simulink model "point_Dynamics_a"  (R2018a)
settings: Solver=ode45  StartTime=0.0  StopTime=30  RelTol=1e-6  AbsTol=1e-6
values from neighbouring files (symbols this model uses):
  cableLength = quadrotor.ell    [initSim.m]
  gravity = quadrotor.g    [initSim.m]
  initQuadPos = [1 1 -2]'    [initSim.m]
  loadMass = quadrotor.m    [initSim.m]    (also in quadrotor_dynamics_extended.m = quad.loadMass)
  maxCargoWeight = quadrotor.M/2    [initSim.m]
  quadMass = quadrotor.M    [initSim.m]
  tensionLowerBound = 0.1    [initSim.m]
  tensionUpperBound = 0.1    [initSim.m]
undefined symbols (not defined in the file or in its folder): quadrotor
settings Model: Creator=Henrik  LastModifiedBy=Henrik
settings SolverCC: AutoScaleAbsTol=off  ShapePreserveControl=EnableAll

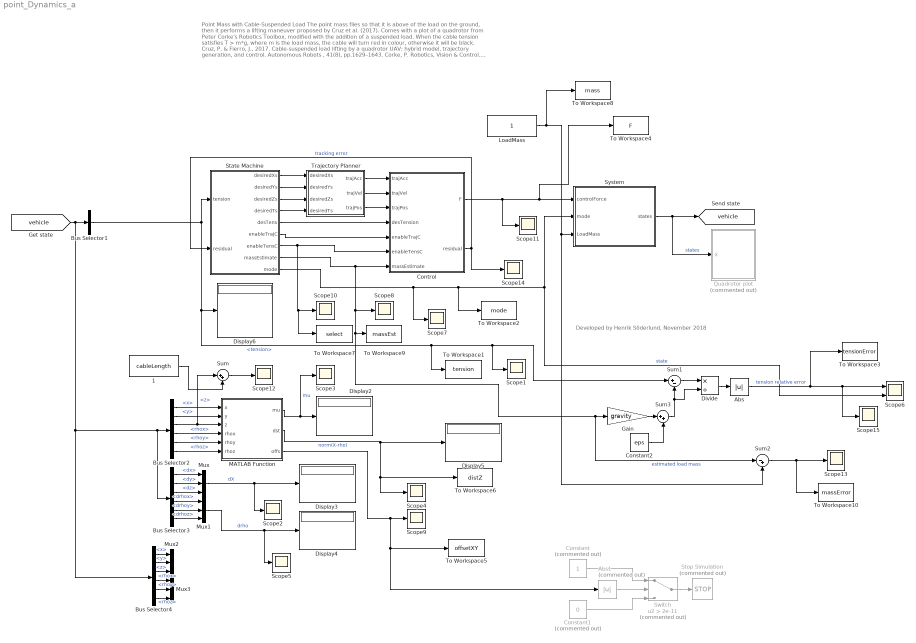
== system point_Dynamics_a ==
  note: Point Mass with Cable-Suspended Load
      |
      | The point mass flies so that it is above of the load on the ground, then it performs a lifting maneuver proposed by Cruz et al. (2017).
      |
      | Comes with a plot of a quadrotor from Peter Corke's Robotics Toolbox, modified with the addition of a suspended load. When the cable tension satisfies T > m*g, where m is the load mass, the cable will turn red in colour, otherwise it will be black.
      |
      | Cruz, P. & Fierro, J., 2017. Cable-suspended load lifting by a quadrotor UAV: hybrid model, trajectory generation, and control. Autonomous Robots , 41(8), pp.1629–1643.
      |
      | Corke, P. Robotics, Vision & Control. Springer (2017).
  note: Developed by Henrik Söderlund, November 2018
  1 : Constant  Value=cableLength
  Abs : Abs
  Abs1 : Abs  Commented=on
  Bus Selector1 : BusSelector  OutputSignals=tension
  Bus Selector2 : BusSelector  OutputSignals=x,y,z,rhox,rhoy,rhoz
  Bus Selector3 : BusSelector  OutputSignals=dx,dy,dz,drhox,drhoy,drhoz
  Bus Selector4 : BusSelector  OutputSignals=x,y,z,rhox,rhoy,rhoz
  Constant : Constant  Commented=on
  Constant1 : Constant  Commented=on  Value=0
  Constant2 : Constant  Value=eps
  Control : Subsystem
  Display{2..6} (5 alike) : Display
  Divide : Product  Inputs=*/
  Gain : Gain  Gain=gravity
  LoadMass : Constant
  MATLAB Function : MATLAB Function  TreatAsAtomicUnit=on
  Mux{,1..3} (4 alike) : Mux  Inputs=3
  Quadrotor plot : Subsystem  Commented=on  AncestorBlock=roblocks/Vehicles/Quadrotor plot  mask{quad=quadrotor, xydim=2, zdim=10}
      mask prompts: quad "Model"; xydim "xy-axes dimension"; zdim "z-axis dimension"
      mask help: Animate quadrotor.
      mask Help:
      | This block graphically displays a quadrotor (flying robot).
      | 
      | A new figure is created and A graphical model of a quadrotor is animated
      | to a pose specified by the state vector input to the block.
      | 
      | The state vector is [x y z roll pitch yaw] in world coordinates and the
      | angles are in radians.
      | 
      | Notes:
      | - The dimensions of the vehicle workspace are set by parameters
  Scope{1..5,7..15} (14 alike) : Scope
  Scope6 : Scope  NumInputPorts=2
  State Machine : Subsystem
  Stop Simulation : Stop  Commented=on
  Sum : Sum  Inputs=|++
  Sum1 : Sum  Inputs=|+-
  Sum2 : Sum  Inputs=|-+
  Sum3 : Sum  Inputs=|++
  Switch : Switch  Commented=on  Criteria=u2 > Threshold  Threshold=2e-11
  System : Subsystem
  To Workspace1 : ToWorkspace  VariableName=tension  SaveFormat=Timeseries  SampleTime=-1
      settings: Save2DSignal=2-D array (concatenate along first dimension)
  To Workspace10 : ToWorkspace  VariableName=massError  SaveFormat=Timeseries  SampleTime=-1
      settings: Save2DSignal=2-D array (concatenate along first dimension)
  To Workspace2 : ToWorkspace  VariableName=mode  SaveFormat=Timeseries  SampleTime=-1
      settings: Save2DSignal=2-D array (concatenate along first dimension)
  To Workspace3 : ToWorkspace  VariableName=tensionError  SaveFormat=Timeseries  SampleTime=-1
      settings: Save2DSignal=2-D array (concatenate along first dimension)
  To Workspace4 : ToWorkspace  VariableName=F  SaveFormat=Timeseries  SampleTime=-1
      settings: Save2DSignal=2-D array (concatenate along first dimension)
  To Workspace5 : ToWorkspace  VariableName=offsetXY  SaveFormat=Timeseries  SampleTime=-1
      settings: Save2DSignal=2-D array (concatenate along first dimension)
  To Workspace6 : ToWorkspace  VariableName=distZ  SaveFormat=Timeseries  SampleTime=-1
      settings: Save2DSignal=2-D array (concatenate along first dimension)
  To Workspace7 : ToWorkspace  VariableName=select  SaveFormat=Timeseries  SampleTime=-1
      settings: Save2DSignal=2-D array (concatenate along first dimension)
  To Workspace8 : ToWorkspace  VariableName=mass  SaveFormat=Timeseries  SampleTime=-1
      settings: Save2DSignal=2-D array (concatenate along first dimension)
  To Workspace9 : ToWorkspace  VariableName=massEst  SaveFormat=Timeseries  SampleTime=-1
      settings: Save2DSignal=2-D array (concatenate along first dimension)
  Trajectory Planner : Subsystem
  tag scope: vehicle=global
  wires:
  [vehicle] -> Bus Selector4/1, Bus Selector2/1, Bus Selector3/1, Bus Selector1/1
  Bus Selector1/1 -> To Workspace1/1, Scope1/1, Sum1/1, Display6/1, State Machine/1(tension)  "<tension>"
  State Machine/1(desiredXs) -> Trajectory Planner/1(desiredXs)
  State Machine/2(desiredYs) -> Trajectory Planner/2(desiredYs)
  State Machine/3(desiredZs) -> Trajectory Planner/3(desiredZs)
  State Machine/4(desiredTs) -> Trajectory Planner/4(desiredTs)
  System/1(states) -> Quadrotor plot/1(X), [vehicle]  "states"
  State Machine/9(mode) -> Scope7/1, To Workspace2/1, Scope6/2, System/2(mode)  "state"
  Bus Selector2/1 -> MATLAB Function/1(x)  "<x>"
  Bus Selector2/2 -> MATLAB Function/2(y)  "<y>"
  Bus Selector2/3 -> Sum/1, MATLAB Function/3(z)  "<z>"
  Bus Selector2/4 -> MATLAB Function/4(rhox)  "<rhox>"
  Bus Selector2/5 -> MATLAB Function/5(rhoy)  "<rhoy>"
  Bus Selector2/6 -> MATLAB Function/6(rhoz)  "<rhoz>"
  MATLAB Function/1(mu) -> Scope3/1, Display2/1  "mu"
  Bus Selector3/2 -> Mux/2  "<dy>"
  Bus Selector3/1 -> Mux/1  "<dx>"
  Bus Selector3/3 -> Mux/3  "<dz>"
  Bus Selector3/4 -> Mux1/1  "<drhox>"
  Bus Selector3/5 -> Mux1/2  "<drhoy>"
  Bus Selector3/6 -> Mux1/3  "<drhoz>"
  Mux/1 -> Scope2/1, Display3/1  "dX"
  Mux1/1 -> Scope5/1, Display4/1  "drho"
  MATLAB Function/2(dst) -> To Workspace6/1, Scope4/1, Display5/1  "norm(X-rho)"
  Control/1(F) -> Scope11/1, To Workspace4/1, System/1(controlForce)
  Trajectory Planner/1(trajAcc) -> Control/1(trajAcc)
  Trajectory Planner/2(trajVel) -> Control/2(trajVel)
  Trajectory Planner/3(trajPos) -> Control/3(trajPos)
  State Machine/5(desTens) -> Control/4(desTension)
  State Machine/6(enableTrajC) -> Control/5(enableTrajC)
  State Machine/7(enableTensC) -> To Workspace7/1, Scope10/1, Control/6(enableTensC)
  State Machine/8(massEstimate) -> Sum2/1, Gain/1, To Workspace9/1, Scope8/1, Control/7(massEstimate)  "estimated load mass"
  Sum3/1 -> Divide/2, Sum1/2
  Sum1/1 -> Divide/1
  Divide/1 -> Abs/1
  Abs/1 -> To Workspace3/1, Scope15/1, Scope6/1  "tension relative error"
  MATLAB Function/3(offs) -> Abs1/1, To Workspace5/1, Scope9/1
  LoadMass/1 -> To Workspace8/1, Sum2/2, System/3(LoadMass)
  Sum/1 -> Scope12/1
  1/1 -> Sum/2
  Control/2(residual) -> Scope14/1, State Machine/2(residual)  "tracking error"
  Sum2/1 -> To Workspace10/1, Scope13/1
  Bus Selector4/1 -> Mux2/1  "<x>"
  Bus Selector4/2 -> Mux2/2  "<y>"
  Bus Selector4/3 -> Mux2/3  "<z>"
  Bus Selector4/5 -> Mux3/2  "<rhoy>"
  Bus Selector4/6 -> Mux3/3  "<rhoz>"
  Bus Selector4/4 -> Mux3/1  "<rhox>"
  Switch/1 -> Stop Simulation/1
  Abs1/1 -> Switch/2
  Constant/1 -> Switch/1
  Constant1/1 -> Switch/3
  Gain/1 -> Sum3/1
  Constant2/1 -> Sum3/2

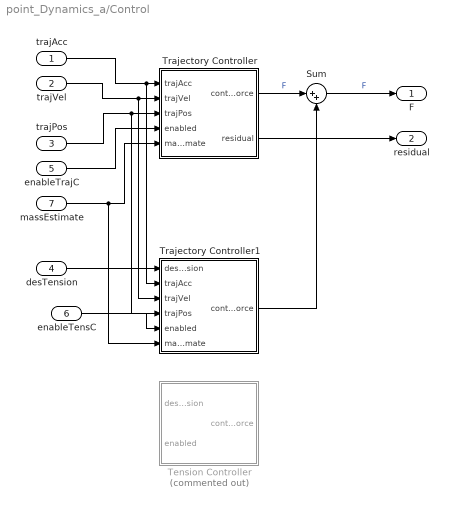
== system point_Dynamics_a/Control ==
  trajAcc : Inport
  trajVel : Inport  Port=2
  trajPos : Inport  Port=3
  desTension : Inport  Port=4
  enableTrajC : Inport  Port=5
  enableTensC : Inport  Port=6
  massEstimate : Inport  Port=7
  Sum : Sum  Inputs=|++
  Tension Controller : Subsystem  Commented=on
  Trajectory Controller : Subsystem
  Trajectory Controller1 : Subsystem
  F : Outport
  residual : Outport  Port=2
  wires:
  Sum/1 -> F/1  "F"
  trajVel/1 -> Trajectory Controller1/3(trajVel), Trajectory Controller/2(trajVel)
  trajPos/1 -> Trajectory Controller1/4(trajPos), Trajectory Controller/3(trajPos)
  enableTrajC/1 -> Trajectory Controller/4(enabled)
  Trajectory Controller/1(controlForce) -> Sum/1  "F"
  trajAcc/1 -> Trajectory Controller1/2(trajAcc), Trajectory Controller/1(trajAcc)
  massEstimate/1 -> Trajectory Controller1/6(massEstimate), Trajectory Controller/5(massEstimate)
  enableTensC/1 -> Trajectory Controller1/5(enabled)
  Trajectory Controller1/1(controlForce) -> Sum/2
  desTension/1 -> Trajectory Controller1/1(desTension)
  Trajectory Controller/2(residual) -> residual/1

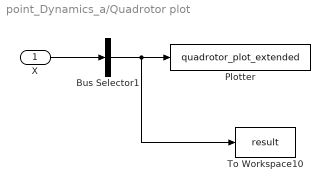
== system point_Dynamics_a/Quadrotor plot ==
  X : Inport
  Bus Selector1 : BusSelector  OutputSignals=x,y,z,yaw,pitch,roll,rhox,rhoy,rhoz,tension  OutputAsBus=on
  Plotter : S-Function  FunctionName=quadrotor_plot_extended  Parameters=[xydim, zdim], 1, 1,quad  SFunctionDeploymentMode=off  EnableBusSupport=off
  To Workspace10 : ToWorkspace  VariableName=result  SampleTime=-1
      settings: Save2DSignal=2-D array (concatenate along first dimension)
  wires:
  X/1 -> Bus Selector1/1
  Bus Selector1/1 -> To Workspace10/1, Plotter/1

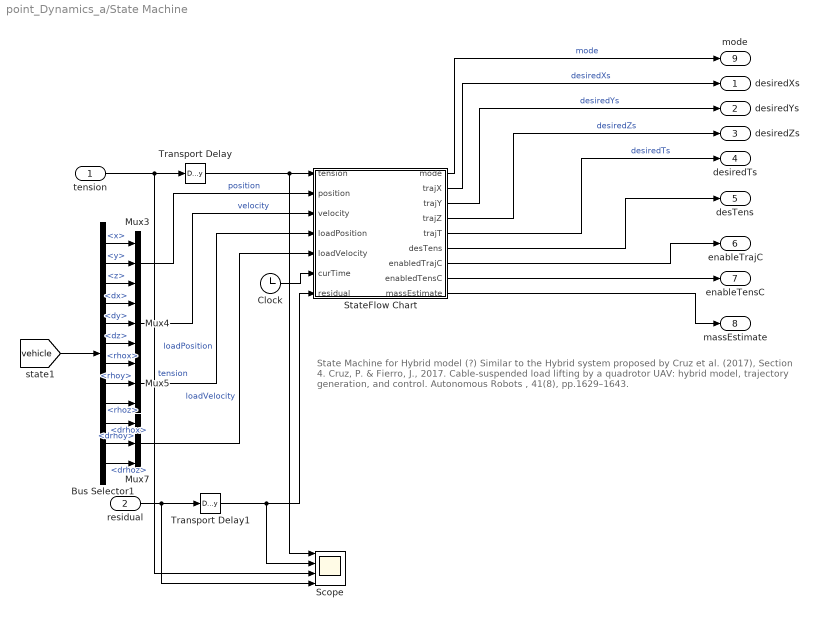
== system point_Dynamics_a/State Machine ==
  note: State Machine for Hybrid model (?)
      |
      | Similar to the Hybrid system proposed by Cruz et al. (2017), Section 4.
      |
      | Cruz, P. & Fierro, J., 2017. Cable-suspended load lifting by a quadrotor UAV: hybrid model, trajectory generation, and control. Autonomous Robots , 41(8), pp.1629–1643.
  tension : Inport
  residual : Inport  Port=2
  Bus Selector1 : BusSelector  OutputSignals=x,y,z,dx,dy,dz,rhox,rhoy,rhoz,drhox,drhoy,drhoz
  Clock : Clock
  Mux{3..5,7} (4 alike) : Mux  Inputs=3
  Scope : Scope  NumInputPorts=4
  StateFlow Chart : Stateflow chart  TreatAsAtomicUnit=on
  Transport Delay : TransportDelay  DelayTime=0.001
  Transport Delay1 : TransportDelay  DelayTime=0.001
  desiredXs : Outport
  desiredYs : Outport  Port=2
  desiredZs : Outport  Port=3
  desiredTs : Outport  Port=4
  desTens : Outport  Port=5
  enableTrajC : Outport  Port=6
  enableTensC : Outport  Port=7
  massEstimate : Outport  Port=8
  mode : Outport  Port=9
  wires:
  StateFlow Chart/5(trajT) -> desiredTs/1  "desiredTs"
  Bus Selector1/1 -> Mux3/1  "<x>"
  Mux3/1 -> StateFlow Chart/2(position)  "position"
  Mux4/1 -> StateFlow Chart/3(velocity)  "velocity"
  Bus Selector1/2 -> Mux3/2  "<y>"
  Mux5/1 -> StateFlow Chart/4(loadPosition)  "loadPosition"
  StateFlow Chart/1(mode) -> mode/1  "mode"
  [vehicle] -> Bus Selector1/1
  Mux7/1 -> StateFlow Chart/5(loadVelocity)  "loadVelocity"
  Bus Selector1/3 -> Mux3/3  "<z>"
  Bus Selector1/7 -> Mux5/1  "<rhox>"
  Bus Selector1/8 -> Mux5/2  "<rhoy>"
  Bus Selector1/9 -> Mux5/3  "<rhoz>"
  Bus Selector1/5 -> Mux4/2  "<dy>"
  Bus Selector1/6 -> Mux4/3  "<dz>"
  Bus Selector1/4 -> Mux4/1  "<dx>"
  Bus Selector1/11 -> Mux7/2  "<drhoy>"
  Bus Selector1/10 -> Mux7/1  "<drhox>"
  Bus Selector1/12 -> Mux7/3  "<drhoz>"
  StateFlow Chart/2(trajX) -> desiredXs/1  "desiredXs"
  StateFlow Chart/4(trajZ) -> desiredZs/1  "desiredZs"
  StateFlow Chart/3(trajY) -> desiredYs/1  "desiredYs"
  tension/1 -> Transport Delay/1, Scope/3  "tension"
  StateFlow Chart/6(desTens) -> desTens/1
  StateFlow Chart/7(enabledTrajC) -> enableTrajC/1
  StateFlow Chart/8(enabledTensC) -> enableTensC/1
  Transport Delay/1 -> Scope/1, StateFlow Chart/1(tension)
  Clock/1 -> StateFlow Chart/6(curTime)
  StateFlow Chart/9(massEstimate) -> massEstimate/1
  residual/1 -> Transport Delay1/1, Scope/4
  Transport Delay1/1 -> Scope/2, StateFlow Chart/7(residual)

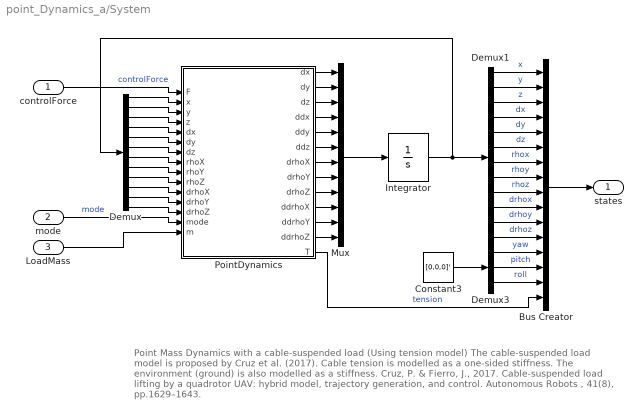
== system point_Dynamics_a/System ==
  note: Point Mass Dynamics with a cable-suspended load (Using tension model)
      |
      | The cable-suspended load model is proposed by Cruz et al. (2017).
      | Cable tension is modelled as a one-sided stiffness. The environment (ground) is also modelled as a stiffness.
      |
      | Cruz, P. & Fierro, J., 2017. Cable-suspended load lifting by a quadrotor UAV: hybrid model, trajectory generation, and control. Autonomous Robots , 41(8), pp.1629–1643.
  controlForce : Inport
  mode : Inport  Port=2
  LoadMass : Inport  Port=3
  Bus Creator : BusCreator  Inputs=16
  Constant3 : Constant  Value=[0,0,0]'
  Demux : Demux  Outputs=12
  Demux1 : Demux  Outputs=12
  Demux3 : Demux  Outputs=3
  Integrator : Integrator  InitialCondition=[initQuadPos' 0 0 0 initLoadPos' 0 0 0]'
  Mux : Mux  Inputs=12
  PointDynamics : MATLAB Function  TreatAsAtomicUnit=on
  states : Outport
  wires:
  PointDynamics/8(drhoY) -> Mux/8
  Demux/11 -> PointDynamics/12("drhoY ")
  Demux/8 -> PointDynamics/9(rhoY)
  PointDynamics/11(ddrhoY) -> Mux/11
  Demux1/3 -> Bus Creator/3  "z"
  PointDynamics/10(ddrhoX) -> Mux/10
  PointDynamics/7(drhoX) -> Mux/7
  PointDynamics/9(drhoZ) -> Mux/9
  Demux/12 -> PointDynamics/13("drhoZ ")
  Demux1/6 -> Bus Creator/6  "dz"
  Demux/2 -> PointDynamics/3(y)
  Demux1/12 -> Bus Creator/12  "drhoz"
  Integrator/1 -> Demux1/1, Demux/1
  PointDynamics/1(dx) -> Mux/1
  Demux1/7 -> Bus Creator/7  "rhox"
  Demux1/1 -> Bus Creator/1  "x"
  PointDynamics/12(ddrhoZ) -> Mux/12
  Demux3/3 -> Bus Creator/15  "roll"
  PointDynamics/13(T) -> Bus Creator/16  "tension"
  Demux1/8 -> Bus Creator/8  "rhoy"
  Demux/10 -> PointDynamics/11("drhoX ")
  Demux/9 -> PointDynamics/10(rhoZ)
  Constant3/1 -> Demux3/1
  Demux3/2 -> Bus Creator/14  "pitch"
  Demux3/1 -> Bus Creator/13  "yaw"
  Bus Creator/1 -> states/1
  controlForce/1 -> PointDynamics/1(F)  "controlForce"
  Mux/1 -> Integrator/1
  Demux/5 -> PointDynamics/6("dy ")
  PointDynamics/5(ddy) -> Mux/5
  PointDynamics/6(ddz) -> Mux/6
  Demux/6 -> PointDynamics/7("dz ")
  Demux/4 -> PointDynamics/5("dx ")
  Demux/1 -> PointDynamics/2(x)
  PointDynamics/2(dy) -> Mux/2
  Demux/3 -> PointDynamics/4(z)
  Demux1/5 -> Bus Creator/5  "dy"
  Demux1/2 -> Bus Creator/2  "y"
  Demux1/4 -> Bus Creator/4  "dx"
  PointDynamics/3(dz) -> Mux/3
  PointDynamics/4(ddx) -> Mux/4
  Demux/7 -> PointDynamics/8(rhoX)
  Demux1/9 -> Bus Creator/9  "rhoz"
  Demux1/10 -> Bus Creator/10  "drhox"
  Demux1/11 -> Bus Creator/11  "drhoy"
  mode/1 -> PointDynamics/14(mode)  "mode"
  LoadMass/1 -> PointDynamics/15(m)

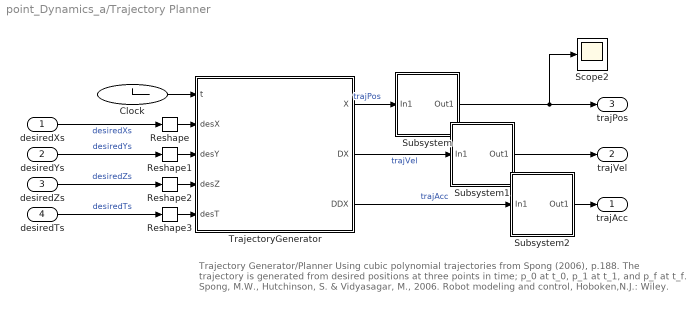
== system point_Dynamics_a/Trajectory Planner ==
  note: Trajectory Generator/Planner
      |
      | Using cubic polynomial trajectories from Spong (2006), p.188.
      |
      | The trajectory is generated from desired positions at three points in time; p_0 at t_0, p_1 at t_1, and p_f at t_f.
      |
      | Spong, M.W., Hutchinson, S. & Vidyasagar, M., 2006. Robot modeling and control, Hoboken,N.J.: Wiley.
  desiredXs : Inport
  desiredYs : Inport  Port=2
  desiredZs : Inport  Port=3
  desiredTs : Inport  Port=4
  Clock : Clock
  Reshape{,1..3} (4 alike) : Reshape  OutputDimensionality=Customize  OutputDimensions=[1,3]
  Scope2 : Scope
  Subsystem : Subsystem
  Subsystem1 : Subsystem
  Subsystem2 : Subsystem
  TrajectoryGenerator : MATLAB Function  TreatAsAtomicUnit=on
  trajAcc : Outport
  trajVel : Outport  Port=2
  trajPos : Outport  Port=3
  wires:
  TrajectoryGenerator/1(X) -> Subsystem/1(In1)  "trajPos"
  Clock/1 -> TrajectoryGenerator/1(t)
  TrajectoryGenerator/2(DX) -> Subsystem1/1(In1)  "trajVel"
  desiredTs/1 -> Reshape3/1  "desiredTs"
  desiredXs/1 -> Reshape/1  "desiredXs"
  TrajectoryGenerator/3(DDX) -> Subsystem2/1(In1)  "trajAcc"
  desiredYs/1 -> Reshape1/1  "desiredYs"
  desiredZs/1 -> Reshape2/1  "desiredZs"
  Reshape/1 -> TrajectoryGenerator/2(desX)
  Reshape1/1 -> TrajectoryGenerator/3(desY)
  Reshape2/1 -> TrajectoryGenerator/4(desZ)
  Reshape3/1 -> TrajectoryGenerator/5(desT)
  Subsystem/1(Out1) -> Scope2/1, trajPos/1
  Subsystem1/1(Out1) -> trajVel/1
  Subsystem2/1(Out1) -> trajAcc/1

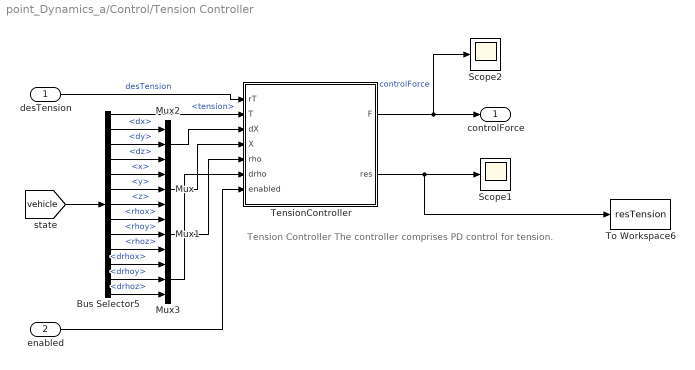
== system point_Dynamics_a/Control/Tension Controller ==
  note: Tension Controller
      |
      | The controller comprises PD control for tension.
  desTension : Inport
  enabled : Inport  Port=2
  Bus Selector5 : BusSelector  OutputSignals=tension,dx,dy,dz,x,y,z,rhox,rhoy,rhoz,drhox,drhoy,drhoz
  Mux{,1..3} (4 alike) : Mux  Inputs=3
  Scope1 : Scope
  Scope2 : Scope
  TensionController : MATLAB Function  TreatAsAtomicUnit=on
  To Workspace6 : ToWorkspace  VariableName=resTension  SaveFormat=Timeseries  SampleTime=-1
      settings: Save2DSignal=2-D array (concatenate along first dimension)
  controlForce : Outport
  wires:
  TensionController/1(F) -> Scope2/1, controlForce/1  "controlForce"
  [vehicle] -> Bus Selector5/1
  desTension/1 -> TensionController/1(rT)  "desTension"
  Bus Selector5/1 -> TensionController/2(T)  "<tension>"
  Bus Selector5/5 -> Mux/1  "<x>"
  Bus Selector5/6 -> Mux/2  "<y>"
  Bus Selector5/7 -> Mux/3  "<z>"
  Mux/1 -> TensionController/4(X)
  Bus Selector5/8 -> Mux1/1  "<rhox>"
  Bus Selector5/9 -> Mux1/2  "<rhoy>"
  Bus Selector5/10 -> Mux1/3  "<rhoz>"
  Mux1/1 -> TensionController/5(rho)
  enabled/1 -> TensionController/7(enabled)
  Bus Selector5/2 -> Mux2/1  "<dx>"
  Bus Selector5/3 -> Mux2/2  "<dy>"
  Bus Selector5/4 -> Mux2/3  "<dz>"
  Mux2/1 -> TensionController/3(dX)
  TensionController/2(res) -> To Workspace6/1, Scope1/1
  Bus Selector5/11 -> Mux3/1  "<drhox>"
  Bus Selector5/12 -> Mux3/2  "<drhoy>"
  Bus Selector5/13 -> Mux3/3  "<drhoz>"
  Mux3/1 -> TensionController/6(drho)

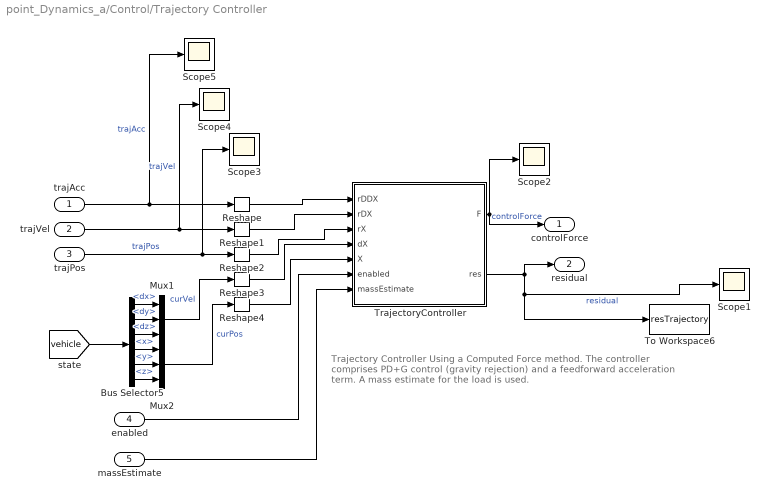
== system point_Dynamics_a/Control/Trajectory Controller ==
  note: Trajectory Controller
      |
      | Using a Computed Force method. The controller comprises PD+G control (gravity rejection) and a feedforward acceleration term.
      |
      | A mass estimate for the load is used.
  trajAcc : Inport
  trajVel : Inport  Port=2
  trajPos : Inport  Port=3
  enabled : Inport  Port=4
  massEstimate : Inport  Port=5
  Bus Selector5 : BusSelector  OutputSignals=dx,dy,dz,x,y,z
  Mux1 : Mux  Inputs=3
  Mux2 : Mux  Inputs=3
  Reshape{,1..4} (5 alike) : Reshape  OutputDimensionality=Column vector (2-D)
  Scope{1..5} (5 alike) : Scope
  To Workspace6 : ToWorkspace  VariableName=resTrajectory  SaveFormat=Timeseries  SampleTime=-1
      settings: Save2DSignal=2-D array (concatenate along first dimension)
  TrajectoryController : MATLAB Function  TreatAsAtomicUnit=on
  controlForce : Outport
  residual : Outport  Port=2
  wires:
  Reshape3/1 -> TrajectoryController/4(dX)
  Bus Selector5/5 -> Mux2/2  "<y>"
  Mux2/1 -> Reshape4/1  "curPos"
  Reshape4/1 -> TrajectoryController/5(X)
  TrajectoryController/1(F) -> controlForce/1, Scope2/1  "controlForce"
  Bus Selector5/3 -> Mux1/3  "<dz>"
  Reshape1/1 -> TrajectoryController/2(rDX)
  Reshape2/1 -> TrajectoryController/3(rX)
  Bus Selector5/1 -> Mux1/1  "<dx>"
  Mux1/1 -> Reshape3/1  "curVel"
  Bus Selector5/4 -> Mux2/1  "<x>"
  Bus Selector5/6 -> Mux2/3  "<z>"
  Bus Selector5/2 -> Mux1/2  "<dy>"
  [vehicle] -> Bus Selector5/1
  trajVel/1 -> Scope4/1, Reshape1/1  "trajVel"
  TrajectoryController/2(res) -> To Workspace6/1, Scope1/1, residual/1  "residual"
  Reshape/1 -> TrajectoryController/1(rDDX)
  trajPos/1 -> Scope3/1, Reshape2/1  "trajPos"
  trajAcc/1 -> Scope5/1, Reshape/1  "trajAcc"
  enabled/1 -> TrajectoryController/6(enabled)
  massEstimate/1 -> TrajectoryController/7(massEstimate)

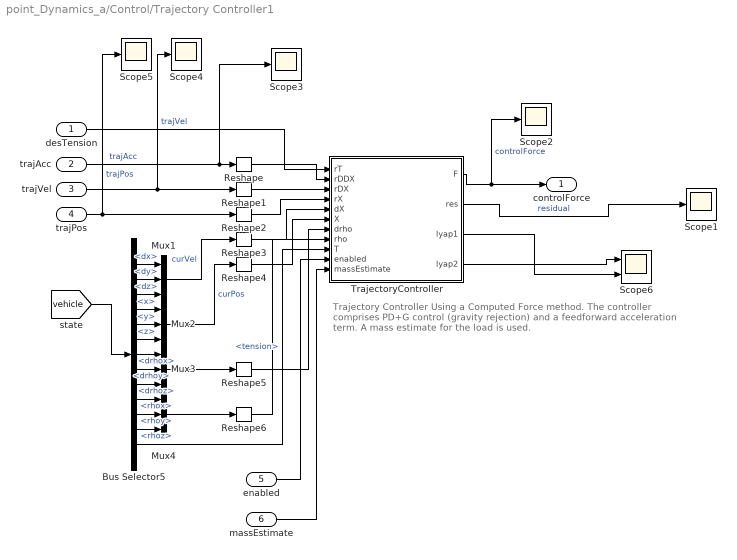
== system point_Dynamics_a/Control/Trajectory Controller1 ==
  note: Trajectory Controller
      |
      | Using a Computed Force method. The controller comprises PD+G control (gravity rejection) and a feedforward acceleration term.
      |
      | A mass estimate for the load is used.
  desTension : Inport
  trajAcc : Inport  Port=2
  trajVel : Inport  Port=3
  trajPos : Inport  Port=4
  enabled : Inport  Port=5
  massEstimate : Inport  Port=6
  Bus Selector5 : BusSelector  OutputSignals=dx,dy,dz,x,y,z,drhox,drhoy,drhoz,rhox,rhoy,rhoz,tension
  Mux{1..4} (4 alike) : Mux  Inputs=3
  Reshape{,1..6} (7 alike) : Reshape  OutputDimensionality=Column vector (2-D)
  Scope{1..5} (5 alike) : Scope
  Scope6 : Scope  NumInputPorts=2
  TrajectoryController : MATLAB Function  TreatAsAtomicUnit=on
  controlForce : Outport
  wires:
  Reshape3/1 -> TrajectoryController/5(dX)
  Bus Selector5/5 -> Mux2/2  "<y>"
  Mux2/1 -> Reshape4/1  "curPos"
  Reshape4/1 -> TrajectoryController/6(X)
  TrajectoryController/1(F) -> Scope2/1, controlForce/1  "controlForce"
  Bus Selector5/3 -> Mux1/3  "<dz>"
  Reshape1/1 -> TrajectoryController/3(rDX)
  Reshape2/1 -> TrajectoryController/4(rX)
  Bus Selector5/1 -> Mux1/1  "<dx>"
  Mux1/1 -> Reshape3/1  "curVel"
  Bus Selector5/4 -> Mux2/1  "<x>"
  Bus Selector5/6 -> Mux2/3  "<z>"
  Bus Selector5/2 -> Mux1/2  "<dy>"
  [vehicle] -> Bus Selector5/1
  trajVel/1 -> Scope4/1, Reshape1/1  "trajVel"
  TrajectoryController/2(res) -> Scope1/1  "residual"
  Reshape/1 -> TrajectoryController/2(rDDX)
  trajPos/1 -> Scope5/1, Reshape2/1  "trajPos"
  trajAcc/1 -> Scope3/1, Reshape/1  "trajAcc"
  enabled/1 -> TrajectoryController/10(enabled)
  massEstimate/1 -> TrajectoryController/11(massEstimate)
  Bus Selector5/7 -> Mux3/1  "<drhox>"
  Bus Selector5/8 -> Mux3/2  "<drhoy>"
  Bus Selector5/9 -> Mux3/3  "<drhoz>"
  Mux3/1 -> Reshape5/1
  Reshape5/1 -> TrajectoryController/7(drho)
  Bus Selector5/10 -> Mux4/1  "<rhox>"
  Bus Selector5/11 -> Mux4/2  "<rhoy>"
  Bus Selector5/12 -> Mux4/3  "<rhoz>"
  Mux4/1 -> Reshape6/1
  Reshape6/1 -> TrajectoryController/8(rho)
  Bus Selector5/13 -> TrajectoryController/9(T)  "<tension>"
  desTension/1 -> TrajectoryController/1(rT)
  TrajectoryController/4(lyap2) -> Scope6/1
  TrajectoryController/3(lyap1) -> Scope6/2

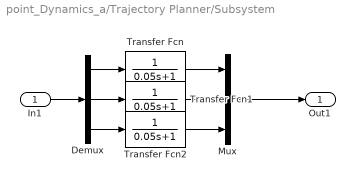
== system point_Dynamics_a/Trajectory Planner/Subsystem ==
  In1 : Inport
  Demux : Demux  Outputs=3
  Mux : Mux  Inputs=3
  Transfer Fcn : TransferFcn  Denominator=[0.05 1]
  Transfer Fcn1 : TransferFcn  Denominator=[0.05 1]
  Transfer Fcn2 : TransferFcn  Denominator=[0.05 1]
  Out1 : Outport
  wires:
  In1/1 -> Demux/1
  Mux/1 -> Out1/1
  Demux/3 -> Transfer Fcn2/1
  Transfer Fcn2/1 -> Mux/3
  Demux/2 -> Transfer Fcn1/1
  Demux/1 -> Transfer Fcn/1
  Transfer Fcn/1 -> Mux/1
  Transfer Fcn1/1 -> Mux/2

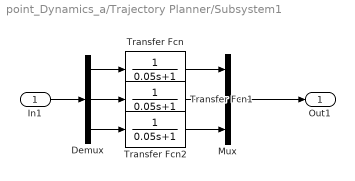
== system point_Dynamics_a/Trajectory Planner/Subsystem1 ==
  In1 : Inport
  Demux : Demux  Outputs=3
  Mux : Mux  Inputs=3
  Transfer Fcn : TransferFcn  Denominator=[0.05 1]
  Transfer Fcn1 : TransferFcn  Denominator=[0.05 1]
  Transfer Fcn2 : TransferFcn  Denominator=[0.05 1]
  Out1 : Outport
  wires:
  In1/1 -> Demux/1
  Mux/1 -> Out1/1
  Demux/3 -> Transfer Fcn2/1
  Transfer Fcn2/1 -> Mux/3
  Demux/2 -> Transfer Fcn1/1
  Demux/1 -> Transfer Fcn/1
  Transfer Fcn/1 -> Mux/1
  Transfer Fcn1/1 -> Mux/2

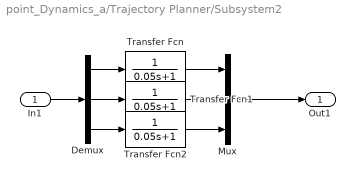
== system point_Dynamics_a/Trajectory Planner/Subsystem2 ==
  In1 : Inport
  Demux : Demux  Outputs=3
  Mux : Mux  Inputs=3
  Transfer Fcn : TransferFcn  Denominator=[0.05 1]
  Transfer Fcn1 : TransferFcn  Denominator=[0.05 1]
  Transfer Fcn2 : TransferFcn  Denominator=[0.05 1]
  Out1 : Outport
  wires:
  In1/1 -> Demux/1
  Mux/1 -> Out1/1
  Demux/3 -> Transfer Fcn2/1
  Transfer Fcn2/1 -> Mux/3
  Demux/2 -> Transfer Fcn1/1
  Demux/1 -> Transfer Fcn/1
  Transfer Fcn/1 -> Mux/1
  Transfer Fcn1/1 -> Mux/2

== matlab function point_Dynamics_a/Control/Trajectory Controller/TrajectoryController ==
  settings: updateMethod=CONTINUOUS
  data: rDDX input; F output; rDX input; rX input; dX input; X input; enabled input; massEstimate input; res output; gravity parameter; loadMass parameter; quadMass parameter
function [F, res]  = trajectoryController(rDDX, rDX, rX, dX, X, enabled, massEstimate, gravity, loadMass, quadMass)

% trajectoryController PD+G control (gravity rejection) and 
%                       a feedforward acceleration term
%
% CALL SEQUENCE: [F, res]=trajectoryController(rDDX, rDX, rX, dX, X)
%
% INPUT:
%   rDDX    desired acceleration (ddot{x}^*, ddot{y}^*, ddot{z}^*)
%   rDX     desired velocity (dot{x}^*, dot{y}^*, dot{z}^*)
%   rX      desired position (x^*, y^*, z^*)
%   DDX     current acceleration (ddot{x}, ddot{y}, ddot{z})
%   DX      current velocity (dot{x}, dot{y}, dot{z})
%   X       current position (x, y, z)
%
% OUTPUT:
%   F       computed output forces (f_x, f_y, f_z)
%   res     residual/error of positions

% PROGRAMMING by Henrik Soderlund (henrik.soderlund@umu.se)
%  2018-11-21 Initial programming

M = quadMass;
m = massEstimate;%loadMass;
g = gravity;

% Define control gains
p = 4;
Kp = p^2;
Kd = 2*p;

% Define direction of gravity.
e3 = [0 0 -1]';

% Define gravity vector.
G = g*e3;

% Compute force using PD+G with feedforward acceleration.
% Scale with M because it makes sense that F=m*a.
if (enabled == 1)
    F = M*(rDDX - Kp*(X - rX) - Kd*(dX - rDX) + G);
else
    F = [0;0;0];
end

% Compute residual.
res = rX - X;

== matlab function point_Dynamics_a/System/PointDynamics ==
  settings: updateMethod=CONTINUOUS
  data: F input; dx output; x input; y input; dy output; z input; dx input; dy input; dz input; rhoX input; rhoY input; rhoZ input; drhoX input; drhoY input; drhoZ input; dz output; ddx output; ddy output; ddz output; mode input; drhoX output; drhoY output; drhoZ output; ddrhoX output; ddrhoY output; ddrhoZ output; T output; gravity parameter; quadMass parameter; m input; cableLength parameter size=1
function [dx,dy,dz,ddx,ddy,ddz,drhoX,drhoY,drhoZ,ddrhoX,ddrhoY,ddrhoZ,T]...
    = pointDynamics ...
    (F,x,y,z,dx,dy,dz,rhoX,rhoY,rhoZ,drhoX,drhoY,drhoZ,mode, gravity, quadMass, m, cableLength) 

% pointDynamics Point mass dynamics with a cable-suspended load.
%
% INPUT:
%   F                   input force vector (f_x, f_y, f_z)
%   x,y,z               position of the point mass at timestep k-1
%   dx,dy,dz            velocity of the point mass at timestep k-1
%   rhoX,rhoY,rhoZ      position of the suspended load at timestep k-1
%   drhoX,drhoY,drhoZ   velocity of the suspended load at timestep k-1
%   T                   tension force of the cable at timestep k-1 [N]
%   mode                current mode of the State Machine (Hybrid system?)
%
% OUTPUT:
%   dx,dy,dz                velocity of the point mass at timestep k
%   ddx,ddy,ddz             accel. of the point mass at timestep k
%   drhoX,drhoY,drhoZ       velocity of the suspended load at timestep k
%   ddrhoX,ddrhoY,ddrhoZ    accel. of the suspended load at timestep k
%   T                       tension force of the cable at timestep k [N]

% PROGRAMMING by Henrik Soderlund (henrik.soderlund@umu.se)
%  2018-11-21 Initial programming

%%%%%%%%%%%%%%%%%%%%%%%%%%%%% BEGIN DEFINES %%%%%%%%%%%%%%%%%%%%%%%%%%%%%%%

M = quadMass;
g = gravity;
ell = cableLength;

% Define direction of gravity.
e3 = [0 0 -1]';

% Define gravity vector.
G = g*e3;

% Define intertia matrix of point mass.
D = M*eye(3);

% Define point mass position as vector
X = [x,y,z]';

% Define point mass velocity as vector
dX = [dx,dy,dz]';

% Define suspended load position as vector
rho = [rhoX, rhoY, rhoZ]';

% Define suspended load velocity as vector
drho = [drhoX, drhoY, drhoZ]';

% Define mu as the vector located at the position of the suspended load,
% pointing in the direction towards the point mass
mu = (X-rho)/norm((X-rho));

%%%%%%%%%%%%%%%%%%%%%%%%%%%%%% END DEFINES %%%%%%%%%%%%%%%%%%%%%%%%%%%%%%%%

%%%%%%%%%%%%%%%%%%%%%%%%%%%% BEGIN DYNAMICS %%%%%%%%%%%%%%%%%%%%%%%%%%%%%%%

% Cable tension is modelled as one-sided stiffness
if (norm(X-rho) >= ell)
    % Spring constant for tension spring model
    ke = 500;
    % Compute the stretch of the cable
    y = norm(X-rho)-ell;
    % Compute tension
    T = m*(ke/ell)*y;
else
    T = 0;
end

% Compute acceleration of point mass
ddX = inv(D)*(F - M*G - T*mu);

% Determine if the load is on the ground or in air.
% The ground is located at z = -0.1.
if (rho(3) >= -0.1)
    % Compute spring constant for ground, we want high stiffness
    groundP = [rho(1:2); 0];
    groundF = 400*norm(rho-groundP);
    
    % Compute acceleration of suspended on ground
    ddrho = (1/m)*T*mu + groundF*e3;
    
    % We have a cable collision at the transition from Setup to Pull
    if (rho(3)+drho(3) < -0.1 && mode == 1)
        disp('COLLISION!');
        
        % Compute inelastic collision impulse
        delta = -m*M*(dX'*mu)/(M+m);
        
        % Update accelerations at instant after collision
        ddX = ddX + (delta/M)*mu;
        ddrho = ddrho - (delta/m)*mu;
    end
else
    % Compute acceleration of suspended load above ground
    ddrho = (1/m)*T*mu - G;
end

% Define output accelerations of point mass
ddx = ddX(1);
ddy = ddX(2);
ddz = ddX(3);

% Define output accelerations of suspended load
ddrhoX = ddrho(1);
ddrhoY = ddrho(2);
ddrhoZ = ddrho(3);

%%%%%%%%%%%%%%%%%%%%%%%%%%%%% END DYNAMICS %%%%%%%%%%%%%%%%%%%%%%%%%%%%%%%%

== matlab function point_Dynamics_a/Trajectory Planner/TrajectoryGenerator ==
  settings: updateMethod=CONTINUOUS
  data: t input; X output; DX output; DDX output; desX input; desY input; desZ input; desT input
function [X, DX, DDX] = trajectoryGenerator(t, desX, desY, desZ, desT)

% trajectoryGenerator Generating cubic polynomial trajectories
%
% CALL SEQUENCE: [X, DX, DDX] = 
%                   trajectoryGenerator(t, desX, desY, desZ, desT)
%
% INPUT:
%   t        current simulation time [s]
%   desX     1x3 vector of desired x values for p_0, p_1, and p_f
%   desY     1x3 vector of desired y values for p_0, p_1, and p_f
%   desZ     1x3 vector of desired z values for p_0, p_1, and p_f
%   desT     1x3 vector of desired time t_0, t_1, and t_f at each point p_j
%
% OUTPUT:
%   X       position at time t in the generated trajectory (x^*,y^*,z^*)
%   DX      velocity at time t in the generated trajectory 
%               (dot{x}^*, dot{y}^*, dot{z}^*)
%   DDX     acceleration at time t in the generated trajectory 
%               (ddot{x}^*, ddot{y}^*, ddot{z}^*)

% PROGRAMMING by Henrik Soderlund (henrik.soderlund@umu.se)
%  2018-11-01 Initial programming

% Redefine name for 1x3 time interval
t_int = desT;
% Redefine name for 1x3 x interval
x = desX;
% Redefine name for 1x3 y interval
y = desY;
% Redefine name for 1x3 z interval
z = desZ;

% Make sure we do not use the trajectory beyond the final time t_f
if (t <= t_int(3))

% Restructure into matrix form
X_0T = [ x(1), x(2), x(end); 
         y(1), y(2), y(end); 
         z(1), z(2), z(end)];
V_0T = [   0, 0, 0;
           0, 0, 0;
           0, 0, 0];
A_0T = [   0, 0, 0;
           0, 0, 0;
           0, 0, 0];

% Cubic polynomials in matrix form
A_poly = [1, t_int(1), t_int(1)^2, t_int(1)^3, t_int(1)^4, t_int(1)^5;...
          0, 1, 2*t_int(1), 3*t_int(1)^2, 4*t_int(1)^3, 5*t_int(1)^4; ...
          0, 0, 2, 6*t_int(1), 12*t_int(1)^2, 20*t_int(1)^3; ...
          1, t_int(2), t_int(2)^2, t_int(2)^3, t_int(2)^4, t_int(2)^5;...
          0, 1, 2*t_int(2), 3*t_int(2)^2, 4*t_int(2)^3, 5*t_int(2)^4; ...
          0, 0, 2, 6*t_int(2), 12*t_int(2)^2, 20*t_int(2)^3; ...
          1, t_int(3), t_int(3)^2, t_int(3)^3, t_int(3)^4, t_int(3)^5;...
          0, 1, 2*t_int(3), 3*t_int(3)^2, 4*t_int(3)^3, 5*t_int(3)^4; ...
          0, 0, 2, 6*t_int(3), 12*t_int(3)^2, 20*t_int(3)^3]; 
       
% coefficients x
poly_x = A_poly \ [X_0T(1,1); V_0T(1,1); A_0T(1,1); X_0T(1,2); V_0T(1,2); A_0T(1,2); X_0T(1,3); V_0T(1,3); A_0T(1,3)];
poly_x = [poly_x(6), poly_x(5), poly_x(4), poly_x(3), poly_x(2), poly_x(1)];
      
% coefficients y
poly_y = A_poly \ [X_0T(2,1); V_0T(2,1); A_0T(2,1); X_0T(2,2); V_0T(2,2); A_0T(2,2); X_0T(2,3); V_0T(2,3); A_0T(2,3)];
poly_y = [poly_y(6), poly_y(5), poly_y(4), poly_y(3), poly_y(2), poly_y(1)];

% coefficients z
poly_z = A_poly \ [X_0T(3,1); V_0T(3,1); A_0T(3,1); X_0T(3,2); V_0T(3,2); A_0T(3,2); X_0T(3,3); V_0T(3,3); A_0T(3,3)];
poly_z = [poly_z(6), poly_z(5), poly_z(4), poly_z(3), poly_z(2), poly_z(1)];

% Compute trajectory at current time instant
x = polyval(poly_x,t);
y = polyval(poly_y,t);
z = polyval(poly_z,t);
Dx = polyval(polyder(poly_x),t);
Dy = polyval(polyder(poly_y),t);
Dz = polyval(polyder(poly_z),t);
DDx = polyval(polyder(polyder(poly_x)),t);
DDy = polyval(polyder(polyder(poly_y)),t);
DDz = polyval(polyder(polyder(poly_z)),t);

% Store as vectors
X = [x,y,z];
DX = [Dx,Dy,Dz];
DDX = [DDx,DDy,DDz];

else
    
    % Stay at the final position, do not compute velocity and acceleration
    % since we are already at the final position.
    X = [x(3),y(3),z(3)];
    DX = [0,0,0];
    DDX = [0,0,0];

end

== stateflow chart point_Dynamics_a/State Machine/StateFlow Chart ==
  state Init
    entry:
    trajX = [position(1); position(1)/2; 0];
    trajY = [position(2); position(2)/2; 0];
    trajZ = [position(3); -cableLength/4; -cableLength/2];
    trajT = [0; 2.5; 5];
    mode = 0;
    enabledTrajC = 1;
    enabledTensC = 0;
    desTens = 0;
    massEstimate = loadMass;
  note: First, we want to initialise the maneuver by moving the point mass so that we are  straight above the load. We transition to the next state when the point mass has stabilized around the final point of the trajectory
      | [0,0,-cableLength / 2].
  state MoveSetup
    exit:
    trajX = [0; 0; 0];
    trajY = [0; 0; 0];
    trajZ = [position(3); position(3); -cableLength-0.1];
    trajT = [5; 6; 10];
  note: Before we enter the Setup mode, we instruct the point mass to attain a new trajectory. Now we want to move so that the distance between the point mass and the suspended load is more than or equal to the length of the cable. We move on to Setup mode directly.
  state Setup
    entry: mode = 0;
  note: We are now in Setup mode. We wait until the distance between the point mass and the suspended load is more than or equal to the length of the cable.
  state LoadTooLight
    entry:
    mode = 3;
    enabledTrajC = 0;
    enabledTensC = 1;
    trajX = [0; 0; 0];
    trajY = [0; 0; 0];
    trajZ = [position(3); -cableLength; -cableLength/2];
    trajT = [curTime; curTime+5; curTime+10];
  note: We are now in Pull mode. We wait until the tension force is larger than the gravitational pull holding down the load to the ground. We transition back to Setup mode if the tension force of the cable is zero.
      |
      | We disable the trajectory controller and enable the tension controller.
  state Pull
    entry:
    mode = 1;
    enabledTrajC = 0;
    enabledTensC = 1;
    trajX = [0; 0; 0];
    trajY = [0; 0; 0];
    trajZ = [position(3); -cableLength-0.3; -cableLength-0.4];
    trajT = [curTime; (curTime+3+curTime)/2; curTime+3];
    desTens = massEstimate*gravity;
    prevTime = curTime;
  state MoveRaise
    exit:
    trajX = [0; 0; 0];
    trajY = [0; 0; 0];
    trajZ = [position(3); -cableLength-2; -cableLength-4];
    trajT = [curTime; (curTime+5+curTime)/2; curTime+5];
    enabledTrajC = 0;
    enabledTensC = 1;
  note: Before we enter the Raise mode, we instruct the point mass to attain a new trajectory. Now we want to move to the desired height above the ground. We move on to Raise mode directly.
      |
      | We disable the tension controller and enable the trajectory controller again.
  state UpdateMassEstimate
    entry:
    massEstimate = massEstimate + 0.02*((tension-desTens)/desTens);
    %+ tension/(massEstimate*gravity) - (1+tensionUpperBound);
  state LoadOnGround
    entry:
    enabledTrajC = 1;
    enabledTensC = 0;
  note: We are now in Raise mode. The load is now in the air, suspended by the attached cable. The only way to transition back to Pull mode is if the distance between the point mass and the suspended load is less than or equal to the length of the cable and the velocity of the suspended load is zero.
  state Raise
    entry: mode = 2;
    desTens = massEstimate*gravity;
  state LoadTooHeavy
    entry:
    mode = 4;
    enabledTrajC = 0;
    enabledTensC = 1;
    trajX = [0; 0; 0];
    trajY = [0; 0; 0];
    trajZ = [position(3); -cableLength; -cableLength/2];
    trajT = [curTime; curTime+5; curTime+10];
  (default) -> Init
  Init -> MoveSetup : [norm(velocity) < 0.1 && norm(residual) < 0.1]
  MoveSetup -> Setup
  Pull -> Setup [order 2] : [abs(tension) < eps]
  Setup -> Pull : [norm(position-loadPosition) >= cableLength]
  LoadTooLight -> LoadOnGround : [position(3)+cableLength < -0.2]
  Pull -> LoadTooLight [order 3] : [curTime-prevTime > 1 && tension <= (1-tensionLowerBound)*massEstimate*gravity]
  Pull -> MoveRaise [order 1] : [curTime-prevTime > 1 && tension > (1-tensionLowerBound)*massEstimate*gravity]
  UpdateMassEstimate -> Raise [order 1] : [massEstimate <= maxCargoWeight]
  MoveRaise -> Raise
  LoadTooHeavy -> LoadOnGround : [position(3)+cableLength < -0.2]
  Raise -> UpdateMassEstimate : [abs((tension-desTens)/(desTens)) > 0 ]
  UpdateMassEstimate -> LoadTooHeavy [order 2] : [massEstimate > maxCargoWeight ]
  data: tension input size=1; position input size=3; velocity input size=3; loadPosition input size=3; mode output size=1; loadVelocity input size=3; trajX output size=3; trajY output size=3; trajZ output size=3; trajT output size=3; gravity parameter double; quadMass parameter; loadMass parameter; cableLength parameter; desTens output size=1; enabledTrajC output size=1; enabledTensC output size=1; curTime input size=1; tensionLowerBound parameter size=1; tensionUpperBound parameter size=1; massEstimate output size=1; maxCargoWeight parameter size=1; residual input; prevTime local size=1 =0

== matlab function point_Dynamics_a/MATLAB Function ==
  data: x input; mu output; y input; z input; rhox input; rhoy input; rhoz input; dst output; offs output
function [mu, dst, offs] = fcn(x,y,z,rhox,rhoy,rhoz)

u = [x;y;z];
v = [rhox;rhoy;rhoz];

dst = norm(u-v);
mu = (u-v)/dst;

offs = [rhox;rhoy];

== matlab function point_Dynamics_a/Control/Tension Controller/TensionController ==
  settings: updateMethod=CONTINUOUS
  data: rT input; T input; F output; dX input; X input; rho input; drho input; enabled input; gravity parameter; loadMass parameter; quadMass parameter; cableLength parameter size=1; res output
function [F, res]  = tensionController(rT, T, dX, X, rho, drho, enabled, gravity, loadMass, quadMass, cableLength)

% tensionController 
%
% CALL SEQUENCE: [F, res]=tensionController(rT, T, X, rho, enabled)
%
% INPUT:

%
% OUTPUT:
%   F       computed output forces (f_x, f_y, f_z)
%   res     residual/error of positions

% PROGRAMMING by Henrik Soderlund (henrik.soderlund@umu.se)
%  2018-11-30 Initial programming

M = quadMass;
m = loadMass;
g = gravity;
ell = cableLength;

% Define direction of gravity.
e3 = [0 0 -1]';

% Define gravity vector.
G = g*e3;

mu = (X-rho)/norm(X-rho);

if (enabled == 1)
    % Compute inverse dynamics of tension at Pull mode
    %F = mu*(rT-(M/ell)*norm(dX)^2) + M*G;
    F = mu*(((m+M)/m)*rT - (M/ell)*norm(dX-drho));
    %F = M*G - 10;
else
    F = [0;0;0];
end

res = rT - T;

== matlab function point_Dynamics_a/Control/Trajectory Controller1/TrajectoryController ==
  settings: updateMethod=CONTINUOUS
  data: rT input; rDDX input; F output; rDX input; rX input; dX input; X input; drho input; rho input; T input; enabled input; massEstimate input; res output; lyap1 output; gravity parameter; loadMass parameter; quadMass parameter; cableLength parameter size=1; lyap2 output
function [F, res, lyap1, lyap2]  = trajectoryTensionController(rT, rDDX, rDX, rX, dX, X, drho, rho, T, enabled, massEstimate, gravity, loadMass, quadMass, cableLength)

% trajectoryController PD+G control (gravity rejection) and 
%                       a feedforward acceleration term
%
% CALL SEQUENCE: [F, res]=trajectoryController(rDDX, rDX, rX, dX, X)
%
% INPUT:
%   rDDX    desired acceleration (ddot{x}^*, ddot{y}^*, ddot{z}^*)
%   rDX     desired velocity (dot{x}^*, dot{y}^*, dot{z}^*)
%   rX      desired position (x^*, y^*, z^*)
%   DDX     current acceleration (ddot{x}, ddot{y}, ddot{z})
%   DX      current velocity (dot{x}, dot{y}, dot{z})
%   X       current position (x, y, z)
%
% OUTPUT:
%   F       computed output forces (f_x, f_y, f_z)
%   res     residual/error of positions

% PROGRAMMING by Henrik Soderlund (henrik.soderlund@umu.se)
%  2018-11-21 Initial programming

M = quadMass;
m = massEstimate;%loadMass;
g = gravity;
ell = cableLength;

% Define control gains
p = 4;
Kp = p^2;
Kd = 2*p;

Lambda = 10;

% Define direction of gravity.
e3 = [0 0 -1]';

% Define gravity vector.
G = g*e3;

mu = (X-rho)/norm(X-rho);

% Compute force using PD+G with feedforward acceleration.
% Scale with M because it makes sense that F=m*a.
if (enabled == 1)
    F = M*(rDDX - Kp*(X - rX) - Kd*(dX - rDX) + G) + (T - m*Lambda*(T - rT))*mu;
    
    %F = M*(rDDX - Kp*(X - rX) + G) + (T - m*Lambda*(T - rT))*mu;

    %hatM = m/(M+m);
    %F = M/(1-hatM)*(rDDX - Kp*(X - rX) - Kd*(dX - rDX) + G - ((hatM/ell)*norm(dX-drho)^2)*mu);
    
    %hatM = m/(M+m);
    %F = M/(1-hatM)*(rDDX - Kp*(X - rX) - Kd*(dX - rDX) + G - ((hatM/ell)*norm(dX-drho)^2)*mu) - m*Lambda*(T - rT)*mu;
    
    %F = (M+m)*(rDDX - Kp*(X - rX) - Kd*(dX - rDX) + G);
    
    %hatM = m/(M+m);
    %F = (M/(1-hatM+m*Lambda*hatM))*(rDDX - Kp*(X - rX) - Kd*(dX - rDX) ...
    %    + G - ((hatM*(1+m)/ell)*norm(dX-drho)^2)*mu + ...
    %    (m/M)*Lambda*hatM*(T - rT)*mu);
else
    F = [0;0;0];
end

% Compute residual.
res = rX - X;

lyap1 = -(dX - rDX)'*Kd*(dX - rDX) -mu'*(m*Lambda*(T - rT)^2)*mu;
lyap2 = -(dX - rDX)'*Kd*(dX - rDX);
